simulink model "parallel_sum"  (Simulink 7.6)
settings: Solver=ode45  StartTime=0.0  StopTime=10.0  RelTol=1e-3
libraries: simulink x8
settings Model: Creator=Docencia  LastModifiedBy=Docencia

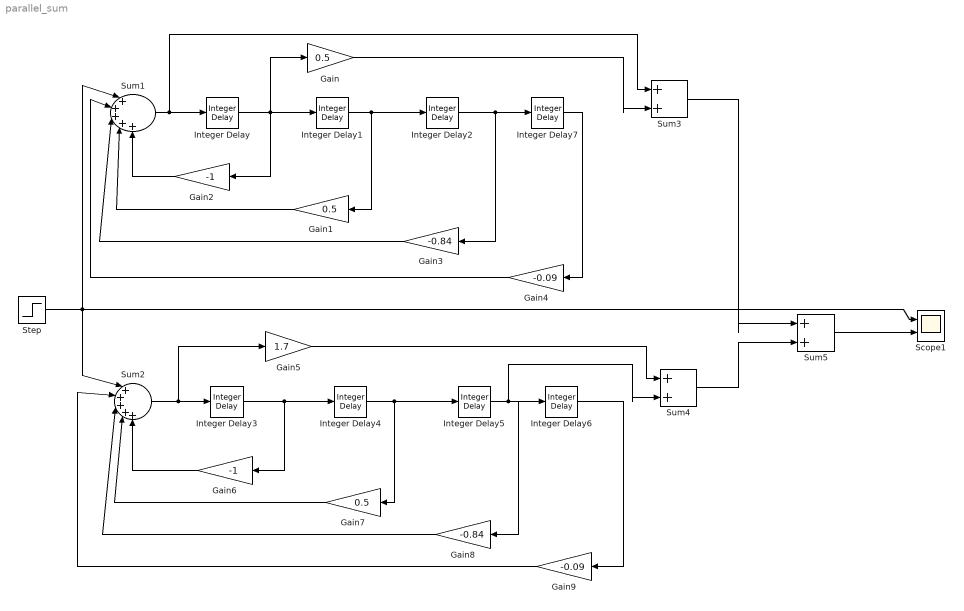
== system parallel_sum ==
  Gain : Gain  Gain=0.5
  Gain1 : Gain  Gain=0.5
  Gain2 : Gain  Gain=-1
  Gain3 : Gain  Gain=-0.84
  Gain4 : Gain  Gain=-0.09
  Gain5 : Gain  Gain=1.7
  Gain6 : Gain  Gain=-1
  Gain7 : Gain  Gain=0.5
  Gain8 : Gain  Gain=-0.84
  Gain9 : Gain  Gain=-0.09
  Integer Delay{,1..7} (8 alike) : simulink/Discrete/Integer Delay  NumDelays=1  vinit=0.0  samptime=-1
  Scope1 : Scope  NumInputPorts=2
      settings: YMin=-5~-5  YMax=5~5
  Step : Step  Time=2  SampleTime=0
  Sum1 : Sum  Inputs=|+++++
  Sum2 : Sum  Inputs=|+++++
  Sum3 : Sum  Inputs=|++
  Sum4 : Sum  Inputs=|++
  Sum5 : Sum  Inputs=|++
  wires:
  Step/1 -> Sum1/1, Sum2/1, Scope1/1
  Sum1/1 -> Integer Delay/1, Sum3/1
  Integer Delay/1 -> Integer Delay1/1, Gain/1, Gain2/1
  Integer Delay1/1 -> Integer Delay2/1, Gain1/1
  Gain/1 -> Sum3/2
  Integer Delay2/1 -> Integer Delay7/1, Gain3/1
  Integer Delay7/1 -> Gain4/1
  Gain4/1 -> Sum1/2
  Gain3/1 -> Sum1/3
  Gain1/1 -> Sum1/4
  Gain2/1 -> Sum1/5
  Sum2/1 -> Integer Delay3/1, Gain5/1
  Integer Delay3/1 -> Integer Delay4/1, Gain6/1
  Integer Delay4/1 -> Integer Delay5/1, Gain7/1
  Gain5/1 -> Sum4/1
  Integer Delay5/1 -> Sum4/2, Integer Delay6/1, Gain8/1
  Integer Delay6/1 -> Gain9/1
  Gain9/1 -> Sum2/2
  Gain8/1 -> Sum2/3
  Gain7/1 -> Sum2/4
  Gain6/1 -> Sum2/5
  Sum3/1 -> Sum5/1
  Sum4/1 -> Sum5/2
  Sum5/1 -> Scope1/2
